simulink model "SquadCopter_Open_Loop"  (R2018a)
settings: Solver=VariableStepAuto  StartTime=0.0  StopTime=10.0  RelTol=1e-3
settings Model: Creator=karee  LastModifiedBy=karee

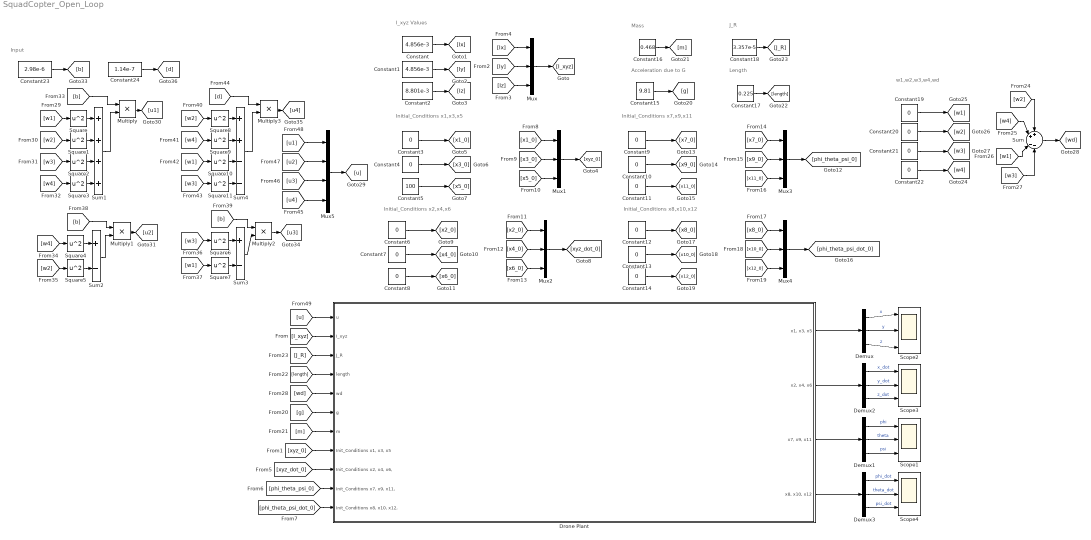
== system SquadCopter_Open_Loop ==
  note: w1,w2,w3,w4,wd
  note: Acceleration due to G
  note: Initial_Conditions x8,x10,x12
  note: Initial_Conditions x7,x9,x11
  note: Initial_Conditions x2,x4,x6
  note: Initial_Conditions x1,x3,x5
  note: I_xyz Values
  note: Mass
  note: Length
  note: J_R
  note: Input
  Constant : Constant  Value=4.856e-3
  Constant1 : Constant  Value=4.856e-3
  Constant{3..4,6..14,19..22} (15 alike) : Constant  Value=0
  Constant15 : Constant  Value=9.81
  Constant16 : Constant  Value=0.468
  Constant17 : Constant  Value=0.225
  Constant18 : Constant  Value=3.357e-5
  Constant2 : Constant  Value=8.801e-3
  Constant23 : Constant  Value=2.98e-6
  Constant24 : Constant  Value=1.14e-7
  Constant5 : Constant  Value=100
  Demux{,1..3} (4 alike) : Demux  Outputs=3
  Drone Plant : Subsystem
  Multiply{,1..3} (4 alike) : Product
  Mux{,1..4} (5 alike) : Mux  Inputs=3
  Mux5 : Mux
  Scope{1..4} (4 alike) : Scope  NumInputPorts=3
  Square{,1..11} (12 alike) : Math  Operator=square  SaturateOnIntegerOverflow=on
  Sum : Sum  Inputs=++|--
  Sum1 : Sum  Inputs=4
  Sum2 : Sum  Inputs=+-
  Sum3 : Sum  Inputs=+-
  Sum4 : Sum  Inputs=++--
  wires:
  [I_xyz] -> Drone Plant/2(I_xyz)
  [xyz_0] -> Drone Plant/8("Init_Conditions x1, x3, x5")
  [Iz] -> Mux/3
  Constant1/1 -> [Iy]
  Constant2/1 -> [Iz]
  [Iy] -> Mux/2
  Constant/1 -> [Ix]
  Mux/1 -> [I_xyz]
  [Ix] -> Mux/1
  [xyz_dot_0] -> Drone Plant/9("Init_Conditions x2, x4, x6,")
  [phi_theta_psi_0] -> Drone Plant/10("Init_Conditions x7, x9, x11,")
  [phi_theta_psi_dot_0] -> Drone Plant/11("Init_Conditions x8, x10, x12,")
  Constant4/1 -> [x3_0]
  [x3_0] -> Mux1/2
  [x5_0] -> Mux1/3
  Constant3/1 -> [x1_0]
  Constant5/1 -> [x5_0]
  Mux1/1 -> [xyz_0]
  [x1_0] -> Mux1/1
  [x2_0] -> Mux2/1
  Mux2/1 -> [xyz_dot_0]
  Constant8/1 -> [x6_0]
  Constant6/1 -> [x2_0]
  [x6_0] -> Mux2/3
  [x4_0] -> Mux2/2
  Constant7/1 -> [x4_0]
  Constant10/1 -> [x9_0]
  [x9_0] -> Mux3/2
  [x11_0] -> Mux3/3
  Constant9/1 -> [x7_0]
  Constant11/1 -> [x11_0]
  Mux3/1 -> [phi_theta_psi_0]
  [x7_0] -> Mux3/1
  [x8_0] -> Mux4/1
  Mux4/1 -> [phi_theta_psi_dot_0]
  Constant14/1 -> [x12_0]
  Constant12/1 -> [x8_0]
  [x12_0] -> Mux4/3
  [x10_0] -> Mux4/2
  Constant13/1 -> [x10_0]
  [g] -> Drone Plant/6(g)
  Constant15/1 -> [g]
  Constant16/1 -> [m]
  [m] -> Drone Plant/7(m)
  Constant17/1 -> [length]
  [length] -> Drone Plant/4(length)
  Constant18/1 -> [J_R]
  [J_R] -> Drone Plant/3(J_R)
  Sum/1 -> [wd]
  [w3] -> Sum/4
  [w4] -> Sum/2
  [w1] -> Sum/3
  [w2] -> Sum/1
  Constant22/1 -> [w4]
  Constant21/1 -> [w3]
  Constant19/1 -> [w1]
  Constant20/1 -> [w2]
  [wd] -> Drone Plant/5(wd)
  [w1] -> Square/1
  [w2] -> Square1/1
  [w4] -> Square3/1
  [w3] -> Square2/1
  [b] -> Multiply/1
  Square/1 -> Sum1/1
  Square1/1 -> Sum1/2
  Square2/1 -> Sum1/3
  Square3/1 -> Sum1/4
  Sum1/1 -> Multiply/2
  Constant23/1 -> [b]
  Multiply/1 -> [u1]
  [b] -> Multiply1/1
  [w2] -> Square5/1
  [w4] -> Square4/1
  Square5/1 -> Sum2/2
  Square4/1 -> Sum2/1
  Multiply1/1 -> [u2]
  Sum2/1 -> Multiply1/2
  Multiply2/1 -> [u3]
  [w3] -> Square6/1
  [w1] -> Square7/1
  [b] -> Multiply2/1
  Sum3/1 -> Multiply2/2
  Square6/1 -> Sum3/1
  Square7/1 -> Sum3/2
  Multiply3/1 -> [u4]
  Sum4/1 -> Multiply3/2
  Square11/1 -> Sum4/4
  Square10/1 -> Sum4/3
  Square9/1 -> Sum4/2
  Square8/1 -> Sum4/1
  [d] -> Multiply3/1
  [w1] -> Square10/1
  [w3] -> Square11/1
  [w4] -> Square9/1
  [w2] -> Square8/1
  Constant24/1 -> [d]
  [u1] -> Mux5/1
  [u2] -> Mux5/2
  [u3] -> Mux5/3
  [u4] -> Mux5/4
  Mux5/1 -> [u]
  [u] -> Drone Plant/1(u)
  Drone Plant/1("x1, x3, x5") -> Demux/1
  Demux/1 -> Scope2/1  "x"
  Demux/2 -> Scope2/2  "y"
  Demux/3 -> Scope2/3  "z"
  Demux1/3 -> Scope1/3  "psi"
  Demux1/2 -> Scope1/2  "theta"
  Demux1/1 -> Scope1/1  "phi"
  Drone Plant/3("x7, x9, x11") -> Demux1/1
  Demux2/3 -> Scope3/3  "z_dot"
  Demux2/2 -> Scope3/2  "y_dot"
  Demux2/1 -> Scope3/1  "x_dot"
  Drone Plant/2("x2, x4, x6") -> Demux2/1
  Drone Plant/4("x8, x10, x12") -> Demux3/1
  Demux3/1 -> Scope4/1  "phi_dot"
  Demux3/2 -> Scope4/2  "theta_dot"
  Demux3/3 -> Scope4/3  "psi_dot"

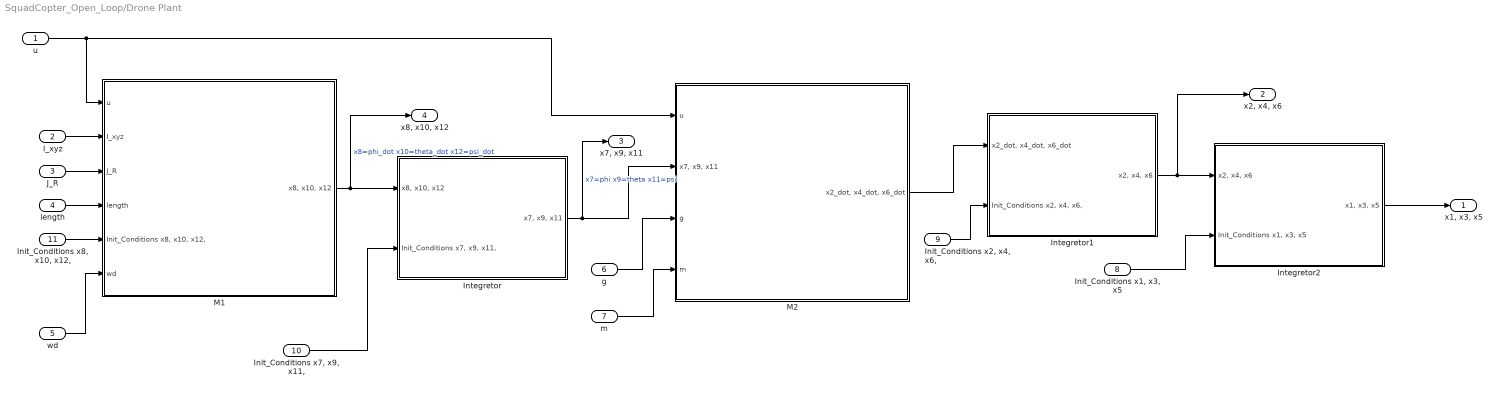
== system SquadCopter_Open_Loop/Drone Plant ==
  u : Inport
  I_xyz : Inport  Port=2
  J_R : Inport  Port=3
  length : Inport  Port=4
  wd : Inport  Port=5
  g : Inport  Port=6
  m : Inport  Port=7
  "Init_Conditions x1, x3, x5" : Inport  Port=8
  "Init_Conditions x2, x4, x6," : Inport  Port=9
  "Init_Conditions x7, x9, x11," : Inport  Port=10
  "Init_Conditions x8, x10, x12," : Inport  Port=11
  Integretor : Subsystem
  Integretor1 : Subsystem
  Integretor2 : Subsystem
  M1 : Subsystem
  M2 : Subsystem
  "x1, x3, x5" : Outport
  "x2, x4, x6" : Outport  Port=2
  "x7, x9, x11" : Outport  Port=3
  "x8, x10, x12" : Outport  Port=4
  wires:
  Integretor2/1("x1, x3, x5") -> "x1, x3, x5"/1
  Integretor1/1("x2, x4, x6") -> "x2, x4, x6"/1, Integretor2/1("x2, x4, x6")
  Integretor/1("x7, x9, x11") -> "x7, x9, x11"/1, M2/2("x7, x9, x11")  "x7=phi x9=theta x11=psi"
  u/1 -> M1/1(u), M2/1(u)
  m/1 -> M2/4(m)
  M1/1("x8, x10, x12") -> "x8, x10, x12"/1, Integretor/1("x8, x10, x12")  "x8=phi_dot x10=theta_dot x12=psi_dot"
  "Init_Conditions x7, x9, x11,"/1 -> Integretor/2("Init_Conditions x7, x9, x11,")
  g/1 -> M2/3(g)
  "Init_Conditions x2, x4, x6,"/1 -> Integretor1/2("Init_Conditions x2, x4, x6,")
  "Init_Conditions x1, x3, x5"/1 -> Integretor2/2("Init_Conditions x1, x3, x5")
  "Init_Conditions x8, x10, x12,"/1 -> M1/5("Init_Conditions x8, x10, x12,")
  length/1 -> M1/4(length)
  M2/1("x2_dot, x4_dot, x6_dot") -> Integretor1/1("x2_dot, x4_dot, x6_dot")
  wd/1 -> M1/6(wd)
  J_R/1 -> M1/3(J_R)
  I_xyz/1 -> M1/2(I_xyz)

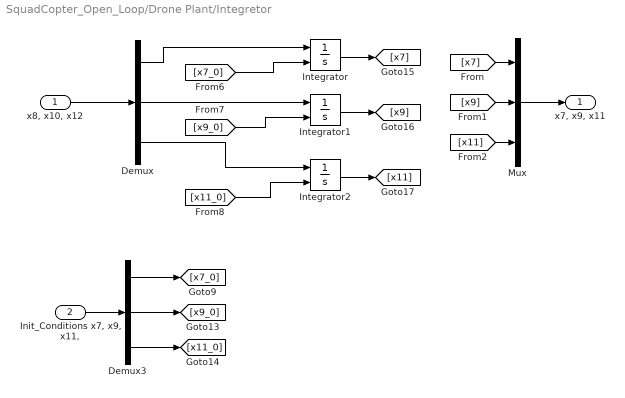
== system SquadCopter_Open_Loop/Drone Plant/Integretor ==
  "x8, x10, x12" : Inport
  "Init_Conditions x7, x9, x11," : Inport  Port=2
  Demux : Demux  Outputs=3
  Demux3 : Demux  Outputs=3
  Integrator : Integrator  InitialConditionSource=external
  Integrator1 : Integrator  InitialConditionSource=external
  Integrator2 : Integrator  InitialConditionSource=external
  Mux : Mux  Inputs=3
  "x7, x9, x11" : Outport
  wires:
  [x7] -> Mux/1
  [x11] -> Mux/3
  Demux3/3 -> [x11_0]
  Integrator2/1 -> [x11]
  [x11_0] -> Integrator2/2
  [x9] -> Mux/2
  "Init_Conditions x7, x9, x11,"/1 -> Demux3/1
  [x7_0] -> Integrator/2
  Mux/1 -> "x7, x9, x11"/1
  [x9_0] -> Integrator1/2
  Integrator/1 -> [x7]
  Demux/1 -> Integrator/1
  Integrator1/1 -> [x9]
  "x8, x10, x12"/1 -> Demux/1
  Demux/2 -> Integrator1/1
  Demux3/2 -> [x9_0]
  Demux3/1 -> [x7_0]
  Demux/3 -> Integrator2/1

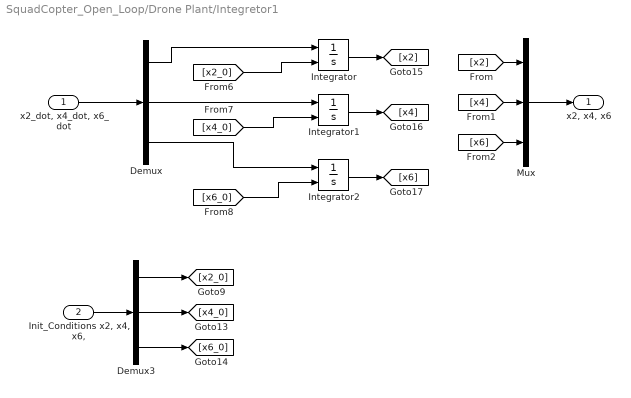
== system SquadCopter_Open_Loop/Drone Plant/Integretor1 ==
  "x2_dot, x4_dot, x6_dot" : Inport
  "Init_Conditions x2, x4, x6," : Inport  Port=2
  Demux : Demux  Outputs=3
  Demux3 : Demux  Outputs=3
  Integrator : Integrator  InitialConditionSource=external
  Integrator1 : Integrator  InitialConditionSource=external
  Integrator2 : Integrator  InitialConditionSource=external
  Mux : Mux  Inputs=3
  "x2, x4, x6" : Outport
  wires:
  Demux/3 -> Integrator2/1
  Demux3/1 -> [x2_0]
  Demux3/2 -> [x4_0]
  Demux/2 -> Integrator1/1
  "x2_dot, x4_dot, x6_dot"/1 -> Demux/1
  Integrator1/1 -> [x4]
  Demux/1 -> Integrator/1
  Integrator/1 -> [x2]
  [x4_0] -> Integrator1/2
  Mux/1 -> "x2, x4, x6"/1
  [x2_0] -> Integrator/2
  "Init_Conditions x2, x4, x6,"/1 -> Demux3/1
  [x4] -> Mux/2
  [x6_0] -> Integrator2/2
  Integrator2/1 -> [x6]
  Demux3/3 -> [x6_0]
  [x6] -> Mux/3
  [x2] -> Mux/1

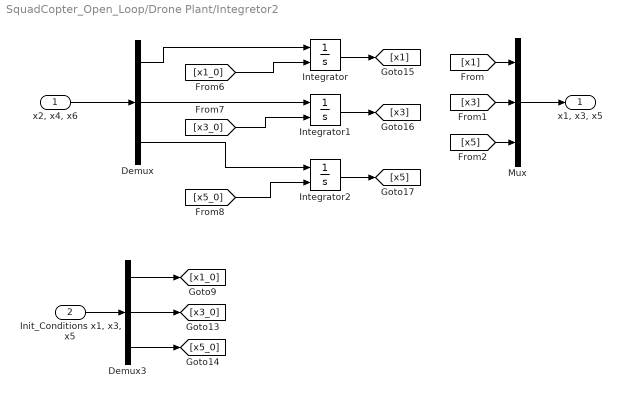
== system SquadCopter_Open_Loop/Drone Plant/Integretor2 ==
  "x2, x4, x6" : Inport
  "Init_Conditions x1, x3, x5" : Inport  Port=2
  Demux : Demux  Outputs=3
  Demux3 : Demux  Outputs=3
  Integrator : Integrator  InitialConditionSource=external
  Integrator1 : Integrator  InitialConditionSource=external
  Integrator2 : Integrator  InitialConditionSource=external
  Mux : Mux  Inputs=3
  "x1, x3, x5" : Outport
  wires:
  [x1] -> Mux/1
  [x5] -> Mux/3
  Demux3/3 -> [x5_0]
  Integrator2/1 -> [x5]
  [x5_0] -> Integrator2/2
  [x3] -> Mux/2
  "Init_Conditions x1, x3, x5"/1 -> Demux3/1
  [x1_0] -> Integrator/2
  Mux/1 -> "x1, x3, x5"/1
  [x3_0] -> Integrator1/2
  Integrator/1 -> [x1]
  Demux/1 -> Integrator/1
  Integrator1/1 -> [x3]
  "x2, x4, x6"/1 -> Demux/1
  Demux/2 -> Integrator1/1
  Demux3/2 -> [x3_0]
  Demux3/1 -> [x1_0]
  Demux/3 -> Integrator2/1

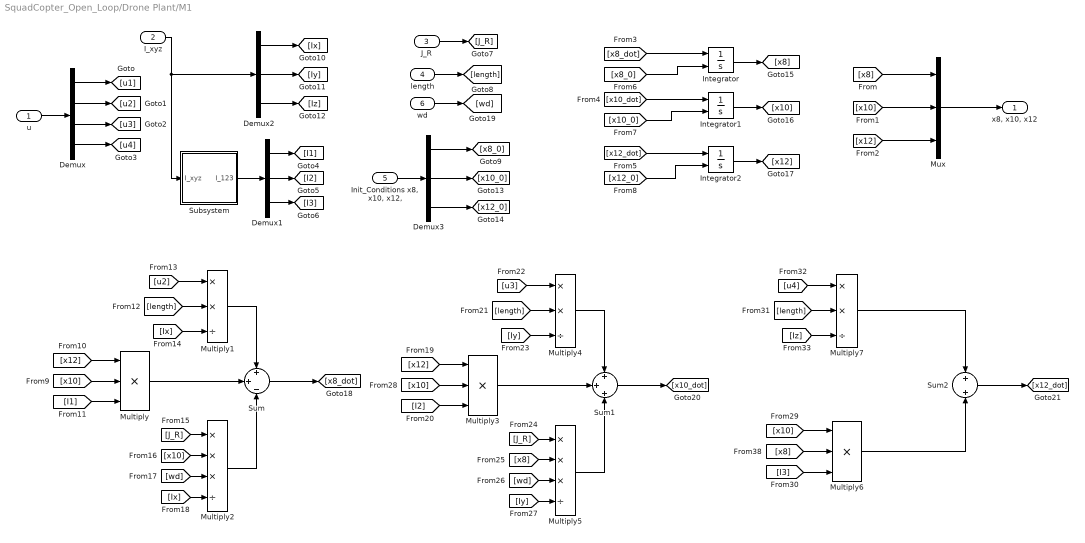
== system SquadCopter_Open_Loop/Drone Plant/M1 ==
  u : Inport
  I_xyz : Inport  Port=2
  J_R : Inport  Port=3
  length : Inport  Port=4
  "Init_Conditions x8, x10, x12," : Inport  Port=5
  wd : Inport  Port=6
  Demux : Demux
  Demux1 : Demux  Outputs=3
  Demux2 : Demux  Outputs=3
  Demux3 : Demux  Outputs=3
  Integrator : Integrator  InitialConditionSource=external
  Integrator1 : Integrator  InitialConditionSource=external
  Integrator2 : Integrator  InitialConditionSource=external
  Multiply : Product  Inputs=3
  Multiply1 : Product  Inputs=**/
  Multiply2 : Product  Inputs=***/
  Multiply3 : Product  Inputs=3
  Multiply4 : Product  Inputs=**/
  Multiply5 : Product  Inputs=***/
  Multiply6 : Product  Inputs=3
  Multiply7 : Product  Inputs=**/
  Mux : Mux  Inputs=3
  Subsystem : Subsystem
  Sum : Sum  Inputs=+|+|-
  Sum1 : Sum  Inputs=+|+|+
  Sum2 : Sum  Inputs=+|+
  "x8, x10, x12" : Outport
  wires:
  u/1 -> Demux/1
  Demux/1 -> [u1]
  Demux/2 -> [u2]
  Demux/3 -> [u3]
  Demux/4 -> [u4]
  Demux2/2 -> [Iy]
  Demux2/3 -> [Iz]
  Demux2/1 -> [Ix]
  I_xyz/1 -> Demux2/1, Subsystem/1(I_xyz)
  Subsystem/1(I_123) -> Demux1/1
  Demux1/1 -> [I1]
  Demux1/2 -> [I2]
  Demux1/3 -> [I3]
  J_R/1 -> [J_R]
  length/1 -> [length]
  "Init_Conditions x8, x10, x12,"/1 -> Demux3/1
  Demux3/1 -> [x8_0]
  Demux3/3 -> [x12_0]
  Demux3/2 -> [x10_0]
  [x10] -> Mux/2
  [x8] -> Mux/1
  [x12] -> Mux/3
  Mux/1 -> "x8, x10, x12"/1
  [x12_dot] -> Integrator2/1
  [x8_dot] -> Integrator/1
  [x10_dot] -> Integrator1/1
  [x8_0] -> Integrator/2
  [x10_0] -> Integrator1/2
  [x12_0] -> Integrator2/2
  Integrator/1 -> [x8]
  Integrator1/1 -> [x10]
  Integrator2/1 -> [x12]
  Sum/1 -> [x8_dot]
  Multiply/1 -> Sum/2
  [x12] -> Multiply/1
  [x10] -> Multiply/2
  [I1] -> Multiply/3
  wd/1 -> [wd]
  [length] -> Multiply1/2
  [u2] -> Multiply1/1
  [Ix] -> Multiply1/3
  Multiply1/1 -> Sum/1
  [J_R] -> Multiply2/1
  [x10] -> Multiply2/2
  [wd] -> Multiply2/3
  [Ix] -> Multiply2/4
  Multiply2/1 -> Sum/3
  Multiply5/1 -> Sum1/3
  [Iy] -> Multiply5/4
  [wd] -> Multiply5/3
  [x8] -> Multiply5/2
  [J_R] -> Multiply5/1
  Multiply4/1 -> Sum1/1
  [Iy] -> Multiply4/3
  [u3] -> Multiply4/1
  [length] -> Multiply4/2
  [I2] -> Multiply3/3
  [x10] -> Multiply3/2
  [x12] -> Multiply3/1
  Multiply3/1 -> Sum1/2
  Sum1/1 -> [x10_dot]
  Sum2/1 -> [x12_dot]
  Multiply6/1 -> Sum2/2
  [x10] -> Multiply6/1
  [x8] -> Multiply6/2
  [I3] -> Multiply6/3
  [length] -> Multiply7/2
  [u4] -> Multiply7/1
  [Iz] -> Multiply7/3
  Multiply7/1 -> Sum2/1

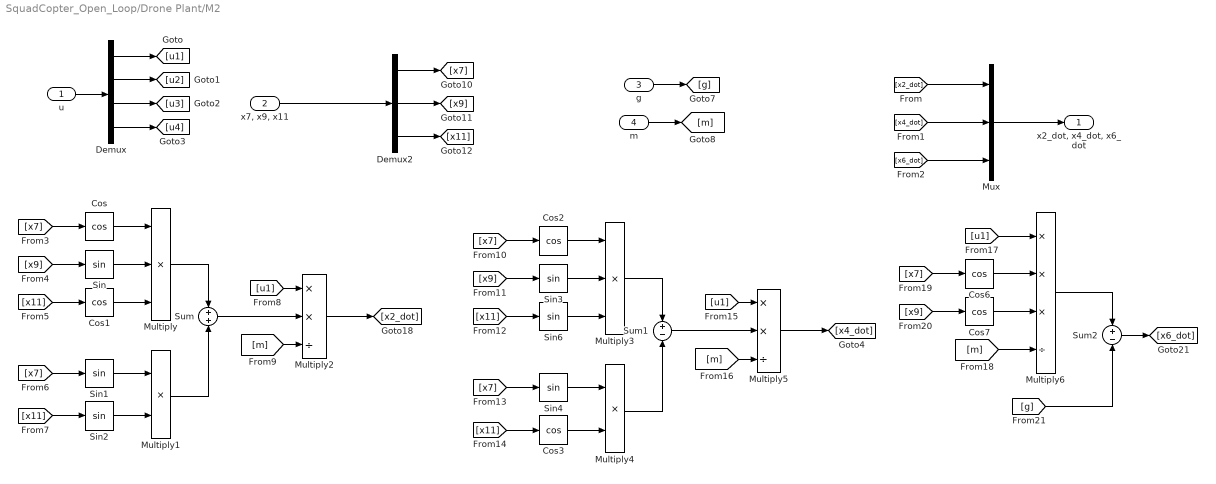
== system SquadCopter_Open_Loop/Drone Plant/M2 ==
  u : Inport
  "x7, x9, x11" : Inport  Port=2
  g : Inport  Port=3
  m : Inport  Port=4
  Cos{,1..3,6..7} (6 alike) : Trigonometry  Operator=cos
  Demux : Demux
  Demux2 : Demux  Outputs=3
  Multiply : Product  Inputs=3
  Multiply1 : Product
  Multiply2 : Product  Inputs=**/
  Multiply3 : Product  Inputs=3
  Multiply4 : Product
  Multiply5 : Product  Inputs=**/
  Multiply6 : Product  Inputs=***/
  Mux : Mux  Inputs=3
  Sin{,1..4,6} (6 alike) : Trigonometry
  Sum : Sum  Inputs=+|+
  Sum1 : Sum  Inputs=+|-
  Sum2 : Sum  Inputs=+|-
  "x2_dot, x4_dot, x6_dot" : Outport
  wires:
  Mux/1 -> "x2_dot, x4_dot, x6_dot"/1
  [x6_dot] -> Mux/3
  [x2_dot] -> Mux/1
  [x4_dot] -> Mux/2
  m/1 -> [m]
  g/1 -> [g]
  Demux/4 -> [u4]
  Demux/3 -> [u3]
  Demux/2 -> [u2]
  Demux/1 -> [u1]
  u/1 -> Demux/1
  "x7, x9, x11"/1 -> Demux2/1
  Demux2/1 -> [x7]
  Demux2/3 -> [x11]
  Demux2/2 -> [x9]
  Multiply/1 -> Sum/1
  Multiply1/1 -> Sum/2
  Sum/1 -> Multiply2/2
  Multiply2/1 -> [x2_dot]
  Sin/1 -> Multiply/2
  Cos/1 -> Multiply/1
  Cos1/1 -> Multiply/3
  [x7] -> Cos/1
  [x9] -> Sin/1
  [x11] -> Cos1/1
  Sin1/1 -> Multiply1/1
  Sin2/1 -> Multiply1/2
  [x7] -> Sin1/1
  [x11] -> Sin2/1
  [u1] -> Multiply2/1
  [m] -> Multiply2/3
  [m] -> Multiply5/3
  [u1] -> Multiply5/1
  [x11] -> Cos3/1
  [x7] -> Sin4/1
  Cos3/1 -> Multiply4/2
  Sin4/1 -> Multiply4/1
  [x11] -> Sin6/1
  [x9] -> Sin3/1
  [x7] -> Cos2/1
  Sin6/1 -> Multiply3/3
  Cos2/1 -> Multiply3/1
  Sin3/1 -> Multiply3/2
  Multiply5/1 -> [x4_dot]
  Sum1/1 -> Multiply5/2
  Multiply4/1 -> Sum1/2
  Multiply3/1 -> Sum1/1
  [x9] -> Cos7/1
  Cos7/1 -> Multiply6/3
  Cos6/1 -> Multiply6/2
  [x7] -> Cos6/1
  [u1] -> Multiply6/1
  [m] -> Multiply6/4
  Multiply6/1 -> Sum2/1
  [g] -> Sum2/2
  Sum2/1 -> [x6_dot]

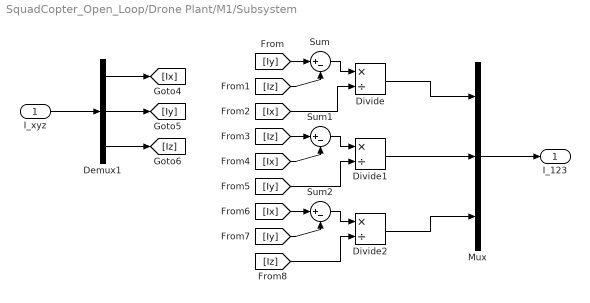
== system SquadCopter_Open_Loop/Drone Plant/M1/Subsystem ==
  I_xyz : Inport
  Demux1 : Demux  Outputs=3
  Divide : Product  Inputs=*/
  Divide1 : Product  Inputs=*/
  Divide2 : Product  Inputs=*/
  Mux : Mux  Inputs=3
  Sum : Sum  Inputs=|+-
  Sum1 : Sum  Inputs=|+-
  Sum2 : Sum  Inputs=|+-
  I_123 : Outport
  wires:
  [Iy] -> Sum2/2
  Divide2/1 -> Mux/3
  [Iy] -> Sum/1
  Sum/1 -> Divide/1
  I_xyz/1 -> Demux1/1
  Sum2/1 -> Divide2/1
  [Ix] -> Sum2/1
  [Iz] -> Divide2/2
  Demux1/3 -> [Iz]
  [Ix] -> Sum1/2
  Demux1/1 -> [Ix]
  [Ix] -> Divide/2
  [Iz] -> Sum/2
  Divide/1 -> Mux/1
  Sum1/1 -> Divide1/1
  Divide1/1 -> Mux/2
  [Iz] -> Sum1/1
  [Iy] -> Divide1/2
  Demux1/2 -> [Iy]
  Mux/1 -> I_123/1
